simulink model "gyroscope_simu"  (R2019a)
settings: Solver=ode3  StartTime=0.0  StopTime=70  FixedStep=Ts  RelTol=1e-3  EnableMultiTasking=on
values from neighbouring files (symbols this model uses):
  A = [0                    0                   0                   1                   0 ... (first row only)    [init_gyroscope.m]
  Aobs = A - L*C    [init_gyroscope.m]
  B = [0                0 ... (first row only)    [init_gyroscope.m]
  C = [1    0   0   0   0 ... (first row only)    [init_gyroscope.m]
  F = Ke(:, 1 : 5)    [init_gyroscope.m]
  g = inv(C*inv(-A + B*K)*B)    [init_gyroscope.m]
  H = Ke(:, 6 : 7)    [init_gyroscope.m]
  K = lqr(A, B, Q, R)    [init_gyroscope.m]
  L = lqr(A', C', W, V)'    [init_gyroscope.m]
libraries: simulink x4
settings Model: ExtModeTrigDuration=100000  Creator=dumonjon  LastModifiedBy=DELL
settings DataIOCC: SaveFormat=StructureWithTime  SignalLoggingSaveFormat=ModelDataLogs  SaveOutput=off  SignalLogging=off  SaveTime=off  ReturnWorkspaceOutputs=off
settings OptimizationCC: ExpressionDepthLimit=2147483647  InitFltsAndDblsToZero=on  LifeSpan=inf
settings DebuggingCC: AlgebraicLoopMsg=none  UnderspecifiedInitializationDetection=Classic  MergeDetectMultiDrivingBlocksExec=none  SolverPrmCheckMsg=warning  FcnCallInpInsideContextMsg=warning  StateNameClashWarn=warning  SFUnexpectedBacktrackingDiag=warning  SFNoUnconditionalDefaultTransitionDiag=warning  SFExecutionAtInitializationDiag=none  ArithmeticOperatorsInVariantConditions=warning
settings HardwareCC: ProdBitPerPointer=32  ProdBitPerSizeT=32  ProdBitPerPtrDiffT=32  ProdLargestAtomicFloat=None  ProdIntDivRoundTo=Undefined  ProdEndianess=Unspecified  ProdWordSize=32  ProdHWDeviceType=32-bit Generic
settings ModelReferenceCC: PropagateSignalLabelsOutOfModel=off
settings SFSimCC: SimUseLocalCustomCode=off  SimParseCustomCode=off
settings RTWCC: SystemTargetFile=rtwin.tlc  TemplateMakefile=rtwin.tmf  Description=Real-Time Windows Target  RTWUseLocalCustomCode=off
settings CodeAppCC: StateflowObjectComments=on
settings TargetCC: ModelReferenceCompliant=off  CompOptLevelCompliant=off  PreserveStateflowLocalDataDimensions=off
settings ConfigComp: CovMetricSettings=dw  CovHtmlReporting=on  CovSaveCumulativeToWorkspaceVar=on  CovSaveSingleToWorkspaceVar=on  CovExternalEMLEnable=off

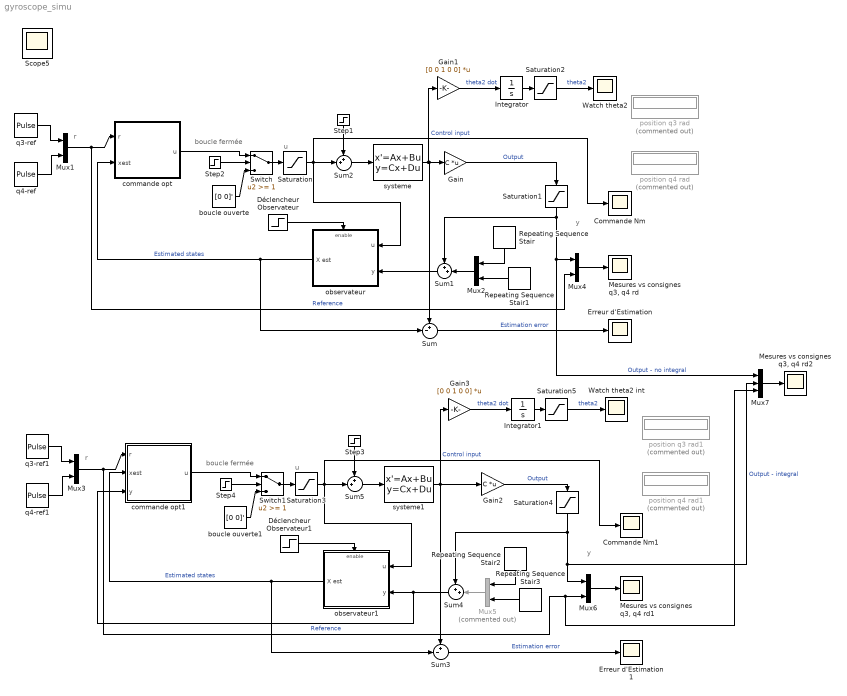
== system gyroscope_simu ==
  note: u
  note: r
  note: y
  note: boucle fermée
  note: u
  note: r
  note: y
  note: boucle fermée
  Commande Nm : Scope
  Commande Nm1 : Scope
  Déclencheur Observateur : Step  SampleTime=0
  Déclencheur Observateur1 : Step  SampleTime=0
  "Erreur d'Estimation " : Scope
  Erreur d'Estimation 1 : Scope
  Gain : Gain  Gain=C  Multiplication=Matrix(K*u) (u vector)
  Gain1 : Gain  Gain=[0 0 1 0 0]  Multiplication=Matrix(K*u) (u vector)
  Gain2 : Gain  Gain=C  Multiplication=Matrix(K*u) (u vector)
  Gain3 : Gain  Gain=[0 0 1 0 0]  Multiplication=Matrix(K*u) (u vector)
  Integrator : Integrator
  Integrator1 : Integrator
  "Mesures vs consignes q3, q4 rd" : Scope
  "Mesures vs consignes q3, q4 rd1" : Scope
  "Mesures vs consignes q3, q4 rd2" : Scope
  Mux{1..4,6} (5 alike) : Mux  Inputs=2
  Mux5 : Mux  Commented=on  Inputs=2
  Mux7 : Mux  Inputs=3
  Repeating Sequence Stair{,1..3} (4 alike) : simulink/Sources/Repeating Sequence Stair  OutValues=[0.8 -0.8].'  tsamp=-1  OutMin=[]  OutMax=[]  OutDataTypeStr=double  OutputDataTypeScalingMode=double  OutDataType=fixdt(0,8)  ConRadixGroup=Best Precision: Vector-wise  OutScaling=2^-12
  Saturation : Saturate  UpperLimit=[0.2 3]  LowerLimit=-[0.2 3]
  Saturation1 : Saturate  UpperLimit=(20*pi/180)*[1 1]  LowerLimit=-(20*pi/180)*[1 1]
  Saturation2 : Saturate  UpperLimit=(20*pi/180)  LowerLimit=-(20*pi/180)
  Saturation3 : Saturate  UpperLimit=[0.2 3]  LowerLimit=-[0.2 3]
  Saturation4 : Saturate  UpperLimit=(20*pi/180)*[1 1]  LowerLimit=-(20*pi/180)*[1 1]
  Saturation5 : Saturate  UpperLimit=(20*pi/180)  LowerLimit=-(20*pi/180)
  Step1 : Step  Time=25  After=0.001  SampleTime=0
  Step2 : Step  Time=15  SampleTime=0
  Step3 : Step  Time=25  After=0.001  SampleTime=0
  Step4 : Step  Time=15  SampleTime=0
  Sum : Sum  Inputs=+-|
  Sum{1..2,4..5} (4 alike) : Sum  Inputs=++|
  Sum3 : Sum  Inputs=+-|
  Switch : Switch  Threshold=1
  Switch1 : Switch  Threshold=1
  Watch theta2 : Scope
  Watch theta2 int : Scope
  boucle ouverte : Constant  Value=[0 0]'
  boucle ouverte1 : Constant  Value=[0 0]'
  commande opt : Subsystem
  commande opt1 : Subsystem
  observateur : Subsystem
  observateur1 : Subsystem
  position q3 rad : Display  Commented=on
  position q3 rad1 : Display  Commented=on
  position q4 rad : Display  Commented=on
  position q4 rad1 : Display  Commented=on
  q3-ref : DiscretePulseGenerator  PulseType=Time based  Amplitude=10*pi/180  Period=20  PulseWidth=50  PhaseDelay=20
  q3-ref1 : DiscretePulseGenerator  PulseType=Time based  Amplitude=10*pi/180  Period=20  PulseWidth=50  PhaseDelay=20
  q4-ref : DiscretePulseGenerator  PulseType=Time based  Amplitude=10*pi/180  Period=20  PulseWidth=50  PhaseDelay=25
  q4-ref1 : DiscretePulseGenerator  PulseType=Time based  Amplitude=10*pi/180  Period=20  PulseWidth=50  PhaseDelay=25
  systeme : StateSpace  A=A  B=B  C=eye(5,5)  D=zeros(5,2)  InitialCondition=0
  systeme1 : StateSpace  A=A  B=B  C=eye(5,5)  D=zeros(5,2)  InitialCondition=0
  Scope5 : Scope
  wires:
  q4-ref/1 -> Mux1/2
  Switch/1 -> Saturation/1
  commande opt/1(u) -> Switch/1
  boucle ouverte/1 -> Switch/3
  Step2/1 -> Switch/2
  q3-ref/1 -> Mux1/1
  Mux4/1 -> "Mesures vs consignes q3, q4 rd"/1
  Mux1/1 -> Mux4/2, commande opt/1(r)  "Reference"
  systeme/1 -> Gain/1, Sum/1, Gain1/1
  Saturation/1 -> Commande Nm/1, Sum2/2, observateur/1(u)  "Control input"
  Saturation1/1 -> Sum1/1, Mux7/1, Mux4/1  "Output - no integral"
  Integrator/1 -> Saturation2/1
  Gain1/1 -> Integrator/1  "theta2 dot"
  Saturation2/1 -> Watch theta2/1  "theta2"
  observateur/1(X est) -> commande opt/2(xest), Sum/2  "Estimated states"
  Sum/1 -> "Erreur d'Estimation "/1  "Estimation error"
  Déclencheur Observateur/1 -> observateur/Enable
  Gain/1 -> Saturation1/1  "Output"
  Sum2/1 -> systeme/1
  Step1/1 -> Sum2/1
  Sum1/1 -> observateur/2(y)
  Mux2/1 -> Sum1/2
  Repeating Sequence Stair/1 -> Mux2/1
  Repeating Sequence Stair1/1 -> Mux2/2
  Gain2/1 -> Saturation4/1  "Output"
  Sum5/1 -> systeme1/1
  Step4/1 -> Switch1/2
  Saturation3/1 -> Commande Nm1/1, Sum5/2, observateur1/1(u)  "Control input"
  Saturation5/1 -> Watch theta2 int/1  "theta2"
  observateur1/1(X est) -> commande opt1/2(xest), Sum3/2  "Estimated states"
  Integrator1/1 -> Saturation5/1
  q3-ref1/1 -> Mux3/1
  commande opt1/1(u) -> Switch1/1
  boucle ouverte1/1 -> Switch1/3
  Switch1/1 -> Saturation3/1
  q4-ref1/1 -> Mux3/2
  Mux5/1 -> Sum4/2
  Mux3/1 -> Mux7/3, Mux6/2, commande opt1/1(r)  "Reference"
  Repeating Sequence Stair2/1 -> Mux5/1
  Repeating Sequence Stair3/1 -> Mux5/2
  Sum4/1 -> commande opt1/3(y), observateur1/2(y)
  Gain3/1 -> Integrator1/1  "theta2 dot"
  Step3/1 -> Sum5/1
  systeme1/1 -> Gain2/1, Sum3/1, Gain3/1
  Déclencheur Observateur1/1 -> observateur1/Enable
  Mux6/1 -> "Mesures vs consignes q3, q4 rd1"/1
  Saturation4/1 -> Sum4/1, Mux6/1, Mux7/2  "Output - integral"
  Sum3/1 -> Erreur d'Estimation 1/1  "Estimation error"
  Mux7/1 -> "Mesures vs consignes q3, q4 rd2"/1

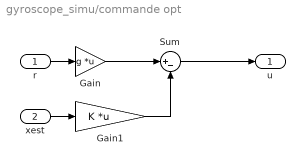
== system gyroscope_simu/commande opt ==
  r : Inport
  xest : Inport  Port=2
  Gain : Gain  Gain=g  Multiplication=Matrix(K*u) (u vector)
  Gain1 : Gain  Gain=K  Multiplication=Matrix(K*u) (u vector)
  Sum : Sum  Inputs=|+-
  u : Outport
  wires:
  r/1 -> Gain/1
  xest/1 -> Gain1/1
  Sum/1 -> u/1
  Gain/1 -> Sum/1
  Gain1/1 -> Sum/2

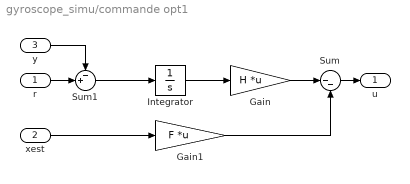
== system gyroscope_simu/commande opt1 ==
  r : Inport
  xest : Inport  Port=2
  y : Inport  Port=3
  Gain : Gain  Gain=H  Multiplication=Matrix(K*u) (u vector)
  Gain1 : Gain  Gain=F  Multiplication=Matrix(K*u) (u vector)
  Integrator : Integrator
  Sum : Sum  Inputs=|--
  Sum1 : Sum  Inputs=-+|
  u : Outport
  wires:
  xest/1 -> Gain1/1
  Sum/1 -> u/1
  Gain/1 -> Sum/1
  Gain1/1 -> Sum/2
  r/1 -> Sum1/2
  y/1 -> Sum1/1
  Sum1/1 -> Integrator/1
  Integrator/1 -> Gain/1

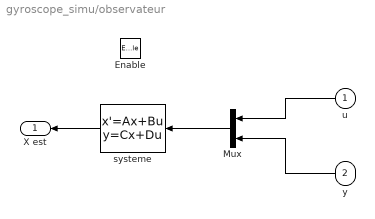
== system gyroscope_simu/observateur ==
  u : Inport
  y : Inport  Port=2
  Enable : EnablePort
  Mux : Mux  Inputs=2
  systeme : StateSpace  A=Aobs  B=[B L]  C=eye(5,5)  D=zeros(5,4)  InitialCondition=0.01
  X est : Outport
  wires:
  systeme/1 -> X est/1
  Mux/1 -> systeme/1
  u/1 -> Mux/1
  y/1 -> Mux/2

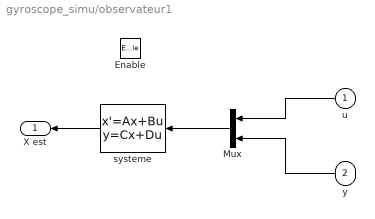
== system gyroscope_simu/observateur1 ==
  u : Inport
  y : Inport  Port=2
  Enable : EnablePort
  Mux : Mux  Inputs=2
  systeme : StateSpace  A=Aobs  B=[B L]  C=eye(5,5)  D=zeros(5,4)  InitialCondition=0.01
  X est : Outport
  wires:
  systeme/1 -> X est/1
  Mux/1 -> systeme/1
  u/1 -> Mux/1
  y/1 -> Mux/2
